simulink model "PendulumRobotArm_OpenLoopslx"  (R2019a)
settings: Solver=VariableStepAuto  StartTime=0.0  StopTime=15  RelTol=1e-3
values from neighbouring files (symbols this model uses):
  c = 1.0791e-5    (= 1.0791e-05)    [Parameters.m]
  g = 9.81    [Parameters.m]
  J = J_motor + m*l^2 + I    (= 0.0704425)    [Parameters.m]
  ke = 50.68*60/(2*pi*1000)    (= 0.483958350954)    [Parameters.m]
  km = 0.415    [Parameters.m]
  l = 3/8    (= 0.375)    [Parameters.m]
  L = 4.8*1e-3    (= 0.0048)    [Parameters.m]
  m = 1/4    (= 0.25)    [Parameters.m]
  R = 9.65    [Parameters.m]
settings Model: Creator=sp_ja  LastModifiedBy=sp_ja

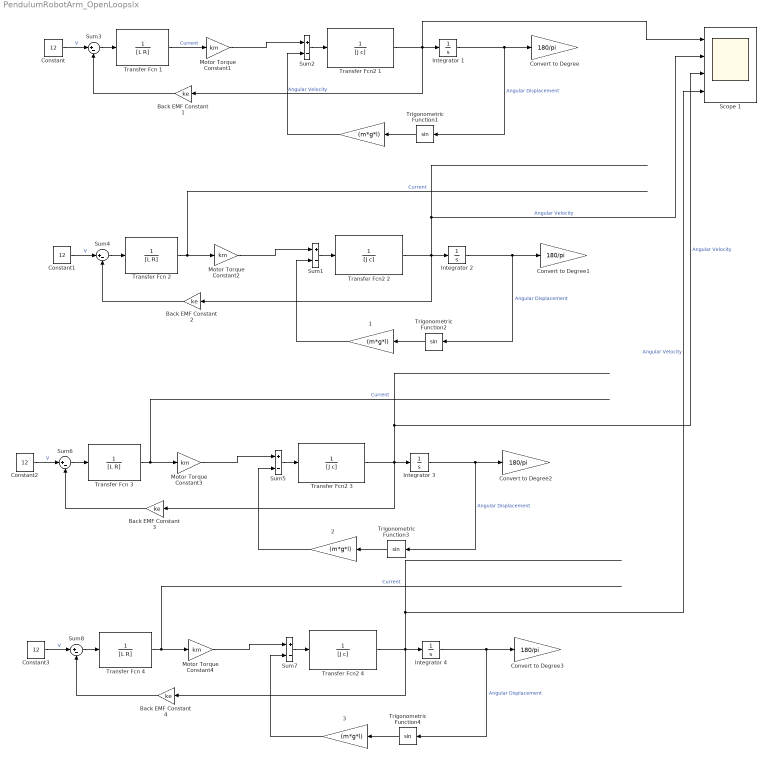
== system PendulumRobotArm_OpenLoopslx ==
    {,1..3} (4 alike) : Gain  Gain=(m*g*l)
    Convert to Degree{,1..3} (4 alike) : Gain  Gain=180/pi
  Back EMF Constant {1..4} (4 alike) : Gain  Gain=ke
  Constant{,1..3} (4 alike) : Constant  Value=12
  Integrator 1 : Integrator  InitialCondition=0*pi/180
  Integrator 2 : Integrator  InitialCondition=30*pi/180
  Integrator 3 : Integrator  InitialCondition=50*pi/180
  Integrator 4 : Integrator  InitialCondition=80*pi/180
  Motor Torque Constant{1..4} (4 alike) : Gain  Gain=km
  Scope 1 : Scope  NumInputPorts=4
  Sum{1..2,5,7} (4 alike) : Sum  Inputs=+-
  Sum{3..4,6,8} (4 alike) : Sum  Inputs=|+-
  Transfer Fcn {1..4} (4 alike) : TransferFcn  Denominator=[L R]
  Transfer Fcn2 {1..4} (4 alike) : TransferFcn  Denominator=[J c]
  Trigonometric Function{1..4} (4 alike) : Trigonometry
  wires:
  Transfer Fcn2 1/1 -> Scope 1/1, Back EMF Constant 1/1, Integrator 1/1  "Angular Velocity"
  Back EMF Constant 1/1 -> Sum3/2
  Sum3/1 -> Transfer Fcn 1/1
  Transfer Fcn 1/1 -> Motor Torque Constant1/1  "Current"
  Constant/1 -> Sum3/1  "V"
  Trigonometric Function1/1 -> "  "/1
  Integrator 1/1 -> Trigonometric Function1/1, "  Convert to Degree"/1  "Angular Displacement"
  "  "/1 -> Sum2/2
  Sum2/1 -> Transfer Fcn2 1/1
  Motor Torque Constant1/1 -> Sum2/1
  Motor Torque Constant2/1 -> Sum1/1
  Constant1/1 -> Sum4/1  "V"
  Trigonometric Function2/1 -> "  1"/1
  Sum1/1 -> Transfer Fcn2 2/1
  "  1"/1 -> Sum1/2
  Integrator 2/1 -> Trigonometric Function2/1, "  Convert to Degree1"/1  "Angular Displacement"
  Transfer Fcn2 2/1 -> Scope 1/2, Back EMF Constant 2/1, Integrator 2/1  "Angular Velocity"
  Sum4/1 -> Transfer Fcn 2/1
  Back EMF Constant 2/1 -> Sum4/2
  Transfer Fcn 2/1 -> Motor Torque Constant2/1  "Current"
  Motor Torque Constant3/1 -> Sum5/1
  Constant2/1 -> Sum6/1  "V"
  Trigonometric Function3/1 -> "  2"/1
  Sum5/1 -> Transfer Fcn2 3/1
  "  2"/1 -> Sum5/2
  Integrator 3/1 -> Trigonometric Function3/1, "  Convert to Degree2"/1  "Angular Displacement"
  Transfer Fcn2 3/1 -> Scope 1/3, Back EMF Constant 3/1, Integrator 3/1  "Angular Velocity"
  Sum6/1 -> Transfer Fcn 3/1
  Back EMF Constant 3/1 -> Sum6/2
  Transfer Fcn 3/1 -> Motor Torque Constant3/1  "Current"
  Back EMF Constant 4/1 -> Sum8/2
  Integrator 4/1 -> Trigonometric Function4/1, "  Convert to Degree3"/1  "Angular Displacement"
  Sum8/1 -> Transfer Fcn 4/1
  Transfer Fcn 4/1 -> Motor Torque Constant4/1  "Current"
  "  3"/1 -> Sum7/2
  Transfer Fcn2 4/1 -> Scope 1/4, Back EMF Constant 4/1, Integrator 4/1  "Angular Velocity"
  Trigonometric Function4/1 -> "  3"/1
  Constant3/1 -> Sum8/1  "V"
  Sum7/1 -> Transfer Fcn2 4/1
  Motor Torque Constant4/1 -> Sum7/1
